simulink model "plant_emulator"  (R2018b)
settings: Solver=FixedStepDiscrete  StartTime=0.0  StopTime=10.0  RelTol=1e-3
settings Model: Creator=jayakumarav  LastModifiedBy=hiterd
settings DebuggingCC: LibraryContextMissingDiagnostic=none
settings SFSimCC: SimUseLocalCustomCode=off
settings RTWCC: RTWUseLocalCustomCode=off

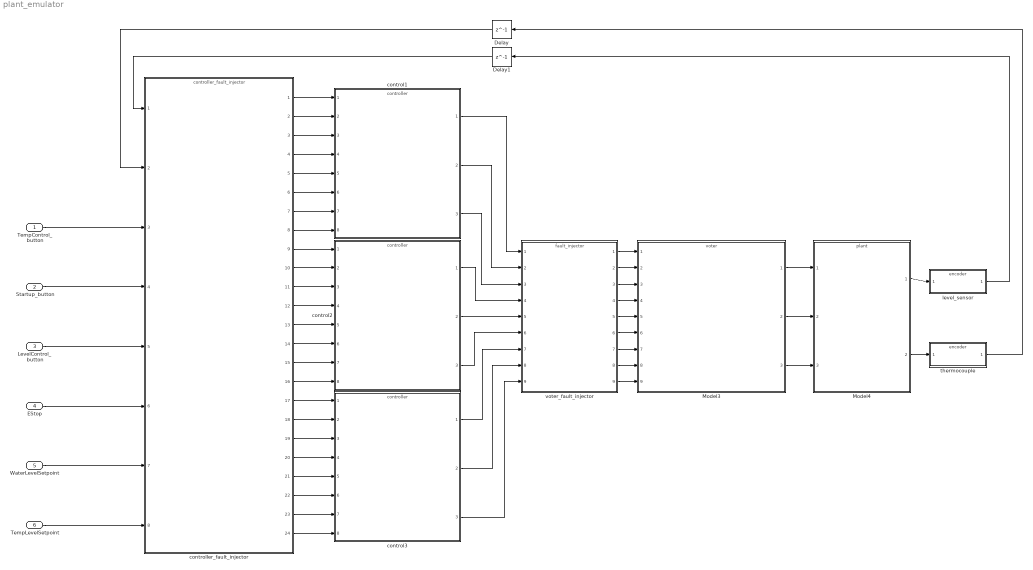
== system plant_emulator ==
  TempControl_button : Inport
  Startup_button : Inport  Port=2
  LevelControl_button : Inport  Port=3
  EStop : Inport  Port=4
  WaterLevelSetpoint : Inport  Port=5
  TempLevelSetpoint : Inport  Port=6
  Delay : Delay  DelayLength=1  InitialCondition=0
  Delay1 : Delay  DelayLength=1  InitialCondition=0
  Model3 : ModelReference  ModelNameDialog=voter.slx  SimulationMode=Normal  ModelReferenceVersion=1.19
  Model4 : ModelReference  ModelNameDialog=plant.slx  SimulationMode=Normal  ModelReferenceVersion=1.19
  control1 : ModelReference  ModelNameDialog=controller.slx  SimulationMode=Normal  ModelReferenceVersion=1.52
  control2 : ModelReference  ModelNameDialog=controller.slx  SimulationMode=Normal  ModelReferenceVersion=1.52
  control3 : ModelReference  ModelNameDialog=controller.slx  SimulationMode=Normal  ModelReferenceVersion=1.52
  controller_fault_injector : ModelReference  ModelNameDialog=controller_fault_injector.slx  SimulationMode=Normal  ModelReferenceVersion=1.13
  level_sensor : ModelReference  ModelNameDialog=encoder.slx  SimulationMode=Normal  ModelReferenceVersion=1.48
  thermocouple : ModelReference  ModelNameDialog=encoder.slx  SimulationMode=Normal  ModelReferenceVersion=1.48
  voter_fault_injector : ModelReference  ModelNameDialog=fault_injector.slx  SimulationMode=Normal  ModelReferenceVersion=1.30
  wires:
  control1/3 -> voter_fault_injector/3
  control1/2 -> voter_fault_injector/2
  control1/1 -> voter_fault_injector/1
  control2/2 -> voter_fault_injector/5
  control2/3 -> voter_fault_injector/6
  control2/1 -> voter_fault_injector/4
  Model3/1 -> Model4/1
  Model3/2 -> Model4/2
  Model3/3 -> Model4/3
  control3/1 -> voter_fault_injector/7
  control3/2 -> voter_fault_injector/8
  control3/3 -> voter_fault_injector/9
  Model4/1 -> level_sensor/1
  Model4/2 -> thermocouple/1
  voter_fault_injector/1 -> Model3/1
  voter_fault_injector/2 -> Model3/2
  voter_fault_injector/3 -> Model3/3
  voter_fault_injector/4 -> Model3/4
  voter_fault_injector/5 -> Model3/5
  voter_fault_injector/6 -> Model3/6
  voter_fault_injector/7 -> Model3/7
  voter_fault_injector/8 -> Model3/8
  voter_fault_injector/9 -> Model3/9
  level_sensor/1 -> Delay1/1
  thermocouple/1 -> Delay/1
  controller_fault_injector/1 -> control1/1
  controller_fault_injector/2 -> control1/2
  controller_fault_injector/3 -> control1/3
  controller_fault_injector/4 -> control1/4
  controller_fault_injector/5 -> control1/5
  controller_fault_injector/6 -> control1/6
  controller_fault_injector/7 -> control1/7
  controller_fault_injector/8 -> control1/8
  controller_fault_injector/9 -> control2/1
  controller_fault_injector/10 -> control2/2
  controller_fault_injector/11 -> control2/3
  controller_fault_injector/12 -> control2/4
  controller_fault_injector/13 -> control2/5
  controller_fault_injector/14 -> control2/6
  controller_fault_injector/15 -> control2/7
  controller_fault_injector/16 -> control2/8
  controller_fault_injector/24 -> control3/8
  controller_fault_injector/23 -> control3/7
  controller_fault_injector/22 -> control3/6
  controller_fault_injector/21 -> control3/5
  controller_fault_injector/20 -> control3/4
  controller_fault_injector/19 -> control3/3
  controller_fault_injector/18 -> control3/2
  controller_fault_injector/17 -> control3/1
  Delay1/1 -> controller_fault_injector/1
  Delay/1 -> controller_fault_injector/2
  TempLevelSetpoint/1 -> controller_fault_injector/8
  WaterLevelSetpoint/1 -> controller_fault_injector/7
  EStop/1 -> controller_fault_injector/6
  LevelControl_button/1 -> controller_fault_injector/5
  Startup_button/1 -> controller_fault_injector/4
  TempControl_button/1 -> controller_fault_injector/3
